simulink model "HW5_model"  (R2021b)
settings: Solver=ode4  StartTime=0.0  StopTime=10  FixedStep=.005  RelTol=1e-3
values from neighbouring files (symbols this model uses):
  C = double(jacobian(out,x_sym))    [HW5.m]
  D2 = ones(6,1)    [HW5.m]
  gamma = sysd.B    [HW5.m]
  K_DT = Z/S    [HW5.m]
  L_DT = P\Y    [HW5.m]
  M_DT = [gamma2, zeros(n,r)]*CB2D2_inv_DT    [HW5.m]
  phi = sysd.A    [HW5.m]
  Ts = .02    (= 0.02)    [HW5.m]
  ue = fsolve(f_xe,[0 0 0]',fsol_opt)    [HW5.m]
  x0 = [.2 .2 .2 0 0 0]'    [HW5.m]
  xe = zeros(6,1)    [HW5.m]
  z0 = zeros(6,1)    [HW5.m]
libraries: vrlib x1
settings Model: Creator=17165  LastModifiedBy=17165

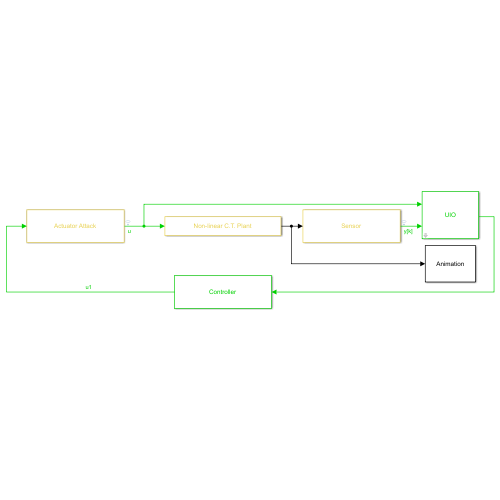
[thumbnail: Simulink's stored preview of the top-level diagram]
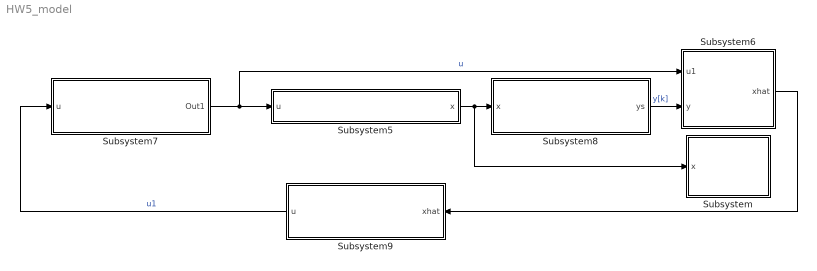
== system HW5_model ==
  Subsystem : Subsystem
      mask Display: disp('Animation')
  Subsystem5 : Subsystem
      mask Display: disp('Non-linear C.T. Plant')
  Subsystem6 : Subsystem  mask{A=phi, B1=gamma, C=C, M=M_DT, L=L_DT}
      mask Display: disp('UIO')
  Subsystem7 : Subsystem
      mask Display: disp('Actuator Attack')
  Subsystem8 : Subsystem
      mask Display: disp('Sensor')
  Subsystem9 : Subsystem
      mask Display: disp('Controller')
  wires:
  Subsystem7/1(Out1) -> Subsystem6/1(u1), Subsystem5/1(u)  "u"
  Subsystem9/1(u) -> Subsystem7/1(u)  "u1"
  Subsystem5/1(x) -> Subsystem/1(x), Subsystem8/1(x)
  Subsystem8/1(ys) -> Subsystem6/2(y)  "y[k]"
  Subsystem6/1(xhat) -> Subsystem9/1(xhat)

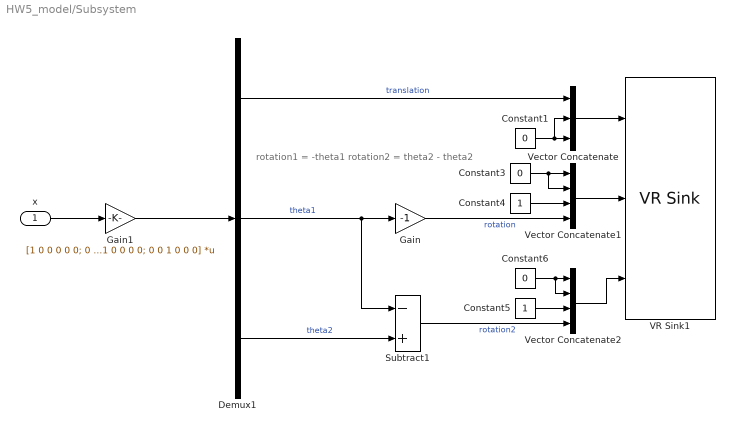
== system HW5_model/Subsystem ==
  note: rotation1 = -theta1
      | rotation2 = theta2 - theta2
  x : Inport
  Constant1 : Constant  Value=0
  Constant3 : Constant  Value=0
  Constant4 : Constant
  Constant5 : Constant
  Constant6 : Constant  Value=0
  Demux1 : Demux  Outputs=3
  Gain : Gain  Gain=-1
  Gain1 : Gain  Gain=[1 0 0 0 0 0; 0 1 0 0 0 0; 0 0 1 0 0 0]  Multiplication=Matrix(K*u)
  Subtract1 : Sum  Inputs=-+
  VR Sink1 : vrlib/VR Sink  InstantiateOnLoad=on  SampleTime=.005  ViewEnable=on  RemoteChange=off  RemoteView=off  FieldsWritten=Cart.translation.3.1.1.double#Rotation1.rotation.4.1.1.double#Rotation2.rotation.4.1.1.double  WorldFileName=DIPC.x3d  AutoView=off  VideoDimensions=[]  AllowVariableSize=off
  Vector Concatenate : Concatenate  NumInputs=3
  Vector Concatenate1 : Concatenate  NumInputs=4
  Vector Concatenate2 : Concatenate  NumInputs=4
  wires:
  Constant3/1 -> Vector Concatenate1/2, Vector Concatenate1/1
  Gain/1 -> Vector Concatenate1/4  "rotation"
  Constant4/1 -> Vector Concatenate1/3
  Constant1/1 -> Vector Concatenate/2, Vector Concatenate/3
  Demux1/2 -> Subtract1/1, Gain/1  "theta1"
  Demux1/3 -> Subtract1/2  "theta2"
  Subtract1/1 -> Vector Concatenate2/4  "rotation2"
  Vector Concatenate1/1 -> VR Sink1/2
  Vector Concatenate2/1 -> VR Sink1/3
  Vector Concatenate/1 -> VR Sink1/1
  Demux1/1 -> Vector Concatenate/1  "translation"
  Constant5/1 -> Vector Concatenate2/3
  Constant6/1 -> Vector Concatenate2/2, Vector Concatenate2/1
  x/1 -> Gain1/1
  Gain1/1 -> Demux1/1

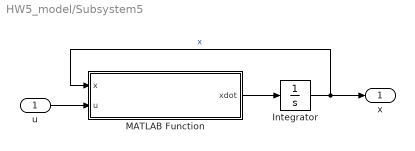
== system HW5_model/Subsystem5 ==
  u : Inport
  Integrator : Integrator  InitialCondition=x0
  MATLAB Function : MATLAB Function  TreatAsAtomicUnit=on
  x : Outport
  wires:
  MATLAB Function/1(xdot) -> Integrator/1
  u/1 -> MATLAB Function/2(u)
  Integrator/1 -> x/1, MATLAB Function/1(x)  "x"

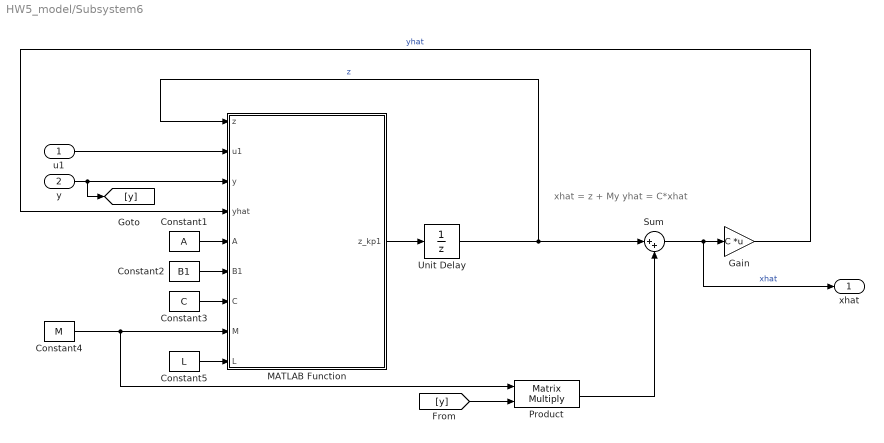
== system HW5_model/Subsystem6 ==
  note: xhat = z + My
      | yhat = C*xhat
  u1 : Inport
  y : Inport  Port=2
  Constant1 : Constant  Value=A
  Constant2 : Constant  Value=B1
  Constant3 : Constant  Value=C
  Constant4 : Constant  Value=M
  Constant5 : Constant  Value=L
  Gain : Gain  Gain=C  Multiplication=Matrix(K*u)
  MATLAB Function : MATLAB Function  TreatAsAtomicUnit=on
  Product : Product  Multiplication=Matrix(*)
  Sum : Sum  Inputs=|++
  Unit Delay : UnitDelay  InitialCondition=z0  SampleTime=Ts  HasFrameUpgradeWarning=on
  xhat : Outport
  wires:
  Constant2/1 -> MATLAB Function/6(B1)
  u1/1 -> MATLAB Function/2(u1)
  Constant3/1 -> MATLAB Function/7(C)
  Constant5/1 -> MATLAB Function/9(L)
  Gain/1 -> MATLAB Function/4(yhat)  "yhat"
  Constant4/1 -> Product/1, MATLAB Function/8(M)
  y/1 -> [y], MATLAB Function/3(y)
  Constant1/1 -> MATLAB Function/5(A)
  Unit Delay/1 -> Sum/1, MATLAB Function/1(z)  "z"
  MATLAB Function/1(z_kp1) -> Unit Delay/1
  [y] -> Product/2
  Product/1 -> Sum/2
  Sum/1 -> xhat/1, Gain/1  "xhat"

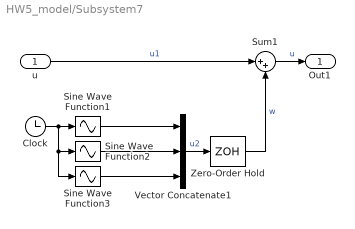
== system HW5_model/Subsystem7 ==
  u : Inport
  Clock : Clock
  Sine Wave Function1 : Sin  TimeSource=Use external signal  Amplitude=.5  Frequency=2*pi  SampleTime=0
  Sine Wave Function2 : Sin  TimeSource=Use external signal  Amplitude=.25  Frequency=4*pi  SampleTime=0
  Sine Wave Function3 : Sin  TimeSource=Use external signal  Amplitude=.25  Frequency=4*pi  SampleTime=0
  Sum1 : Sum  Inputs=|++
  Vector Concatenate1 : Concatenate  NumInputs=3
  Zero-Order Hold : ZeroOrderHold  SampleTime=Ts
  Out1 : Outport
  wires:
  Sine Wave Function1/1 -> Vector Concatenate1/1
  Sine Wave Function2/1 -> Vector Concatenate1/2
  Sine Wave Function3/1 -> Vector Concatenate1/3
  Clock/1 -> Sine Wave Function3/1, Sine Wave Function2/1, Sine Wave Function1/1
  u/1 -> Sum1/1  "u1"
  Vector Concatenate1/1 -> Zero-Order Hold/1  "u2"
  Sum1/1 -> Out1/1  "u"
  Zero-Order Hold/1 -> Sum1/2  "w"

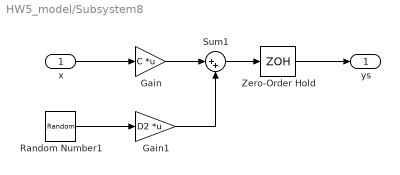
== system HW5_model/Subsystem8 ==
  x : Inport
  Gain : Gain  Gain=C  Multiplication=Matrix(K*u)
  Gain1 : Gain  Gain=D2  Multiplication=Matrix(K*u)
  Random Number1 : RandomNumber  Variance=1e-5
  Sum1 : Sum  Inputs=|++
  Zero-Order Hold : ZeroOrderHold  SampleTime=Ts
  ys : Outport
  wires:
  x/1 -> Gain/1
  Gain/1 -> Sum1/1
  Zero-Order Hold/1 -> ys/1
  Sum1/1 -> Zero-Order Hold/1
  Random Number1/1 -> Gain1/1
  Gain1/1 -> Sum1/2

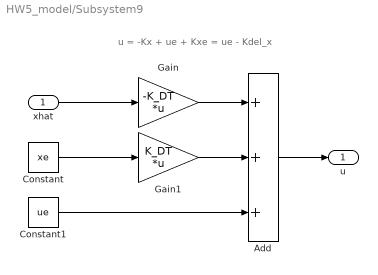
== system HW5_model/Subsystem9 ==
  note: u = -Kx + ue + Kxe = ue - Kdel_x
  xhat : Inport
  Add : Sum  Inputs=+++
  Constant : Constant  Value=xe
  Constant1 : Constant  Value=ue
  Gain : Gain  Gain=-K_DT  Multiplication=Matrix(K*u)
  Gain1 : Gain  Gain=K_DT  Multiplication=Matrix(K*u)
  u : Outport
  wires:
  xhat/1 -> Gain/1
  Gain/1 -> Add/1
  Gain1/1 -> Add/2
  Constant/1 -> Gain1/1
  Constant1/1 -> Add/3
  Add/1 -> u/1

== matlab function HW5_model/Subsystem5/MATLAB Function ==
  data: x input; u input; xdot output
function xdot = DIPC(x, u)

% Define State and Input Vectors
x1          = x(1,1);  % x
x2          = x(2,1);  % theta_1
x3          = x(3,1);  % theta_2
x4          = x(4,1);  % xdot
x5          = x(5,1);  % theta_1_dot
x6          = x(6,1);  % theta_2_dot
u1          = u(1,1);
u2          = u(2,1);
u3          = u(3,1);

% State Dynamics
x1dot       = x4;   % xdot
x2dot       = x5;   % theta_1_dot
x3dot       = x6;   % theta_2_dot

% Numeric Parameters
m1          = 0.5;
L1          = 0.5;
m2          = 0.75;
L2          = 0.75;
M           = 1.5;
g           = 9.81;

% x_ddot
x4dot       = (L2*m2*u2*cos(x2 - 2*x3) - L1*m1*u3*cos(x3) - L2*m2*u2*cos(x2)...
               - L1*m2*u3*cos(x3) - 2*L2*m1*u2*cos(x2) + 2*L1*L2*m1*u1 + L1*L2*m2*u1...
               + L1*m1*u3*cos(2*x2 - x3) + L1*m2*u3*cos(2*x2 - x3) -...
               L1*L2*m2*u1*cos(2*x2 - 2*x3) - L1*L2*g*m1^2*sin(2*x2) +...
               2*L1^2*L2*m1^2*x5^2*sin(x2) - L1*L2*g*m1*m2*sin(2*x2) +...
               L1*L2^2*m1*m2*x6^2*sin(2*x2 - x3) + 2*L1^2*L2*m1*m2*x5^2*sin(x2) +...
               L1*L2^2*m1*m2*x6^2*sin(x3))/(L1*L2*(2*M*m1 + M*m2 + m1*m2 -...
               m1^2*cos(2*x2) + m1^2 - m1*m2*cos(2*x2) - M*m2*cos(2*x2 - 2*x3)));
 
% theta_1_ddot
x5dot       = -(L2*m2*u2*cos(2*x3) - 2*L2*m1*u2 - L2*m2*u2 - 2*L2*M*u2 -...
                2*L1*L2*g*m1^2*sin(x2) + 2*L1*M*u3*cos(x2)*cos(x3) +...
                2*L1*M*u3*sin(x2)*sin(x3) + L1^2*L2*m1^2*x5^2*sin(2*x2) +...
                2*L1*m1*u3*sin(x2)*sin(x3) + 2*L1*m2*u3*sin(x2)*sin(x3) +...
                2*L1*L2*m1*u1*cos(x2) + L1*L2*m2*u1*cos(x2) - 2*L1*L2*M*g*m1*sin(x2)...
                - L1*L2*M*g*m2*sin(x2) - L1*L2*m2*u1*sin(2*x3)*sin(x2) -...
                2*L1*L2*g*m1*m2*sin(x2) + L1^2*L2*m1*m2*x5^2*sin(2*x2) -...
                L1*L2*m2*u1*cos(2*x3)*cos(x2) - L1*L2*M*g*m2*cos(2*x3)*sin(x2) +...
                L1*L2*M*g*m2*sin(2*x3)*cos(x2) - L1^2*L2*M*m2*x5^2*cos(2*x2)*sin(2*x3) +...
                L1^2*L2*M*m2*x5^2*cos(2*x3)*sin(2*x2) - 2*L1*L2^2*M*m2*x6^2*cos(x2)*sin(x3) +...
                2*L1*L2^2*M*m2*x6^2*cos(x3)*sin(x2) + 2*L1*L2^2*m1*m2*x6^2*cos(x3)*sin(x2))/...
                (L1^2*L2*(2*M*m1 + M*m2 + m1*m2 - m1^2*cos(2*x2) + m1^2 -...
                m1*m2*cos(2*x2) - M*m2*cos(2*x2 - 2*x3)));


% theta_2_ddot
x6dot       = (L1*m1^2*u3 + L1*m2^2*u3 - L1*m1^2*u3*cos(2*x2) - L1*m2^2*u3*cos(2*x2) +...
              L2*m2^2*u2*cos(x2 + x3) + 2*L1*M*m1*u3 + 2*L1*M*m2*u3 + 2*L1*m1*m2*u3 -...
              L2*m2^2*u2*cos(x2 - x3) - L2*m1*m2*u2*cos(x2 - x3) - L1*L2*m2^2*u1*cos(x3) -...
              2*L1*m1*m2*u3*cos(2*x2) + L1*L2*m2^2*u1*cos(2*x2 - x3) +...
              L2*m1*m2*u2*cos(x2 + x3) - 2*L2*M*m2*u2*cos(x2 - x3) - L1*L2*m1*m2*u1*cos(x3) +...
              L1*L2*M*g*m2^2*sin(x3) + 2*L1^2*L2*M*m2^2*x5^2*sin(x2 - x3) +...
              L1*L2*m1*m2*u1*cos(2*x2 - x3) + L1*L2^2*M*m2^2*x6^2*sin(2*x2 - 2*x3) -...
              L1*L2*M*g*m2^2*sin(2*x2 - x3) - L1*L2*M*g*m1*m2*sin(2*x2 - x3) +...
              L1*L2*M*g*m1*m2*sin(x3) + 2*L1^2*L2*M*m1*m2*x5^2*sin(x2 - x3))/...
              (L1*L2^2*m2*(2*M*m1 + M*m2 + m1*m2 - m1^2*cos(2*x2) + m1^2 -...
              m1*m2*cos(2*x2) - M*m2*cos(2*x2 - 2*x3)));


xdot        = [x1dot;x2dot;x3dot;x4dot;x5dot;x6dot];

== matlab function HW5_model/Subsystem6/MATLAB Function ==
  data: z input; z_kp1 output; u1 input; y input; yhat input; A input; B1 input; C input; M input; L input
function z_kp1 = UIO(z, u1, y, yhat, A, B1, C, M, L)

z_kp1 = (eye(size(M*C)) - M*C)*(A*z + A*M*y + B1*u1) + L*(y - yhat);

end
